simulink model "formation_with_real_uavs"  (R2022a)
settings: Solver=VariableStepAuto  StartTime=0.0  StopTime=60  RelTol=1e-3
libraries: uavutilslib x1
settings Model: Creator=klebercabral  LastModifiedBy=klebercabral
settings DebuggingCC: UnderSpecifiedDimensionMsg=warning

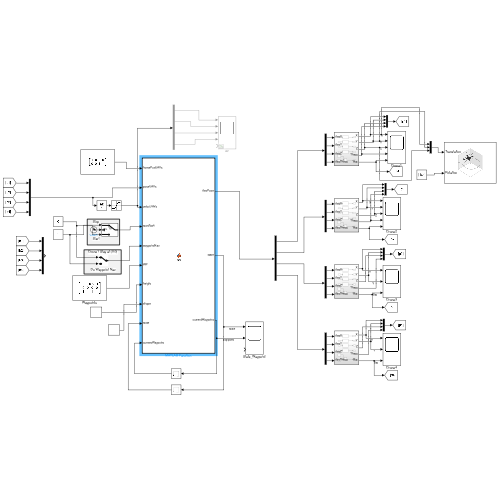
[thumbnail: Simulink's stored preview of the top-level diagram]
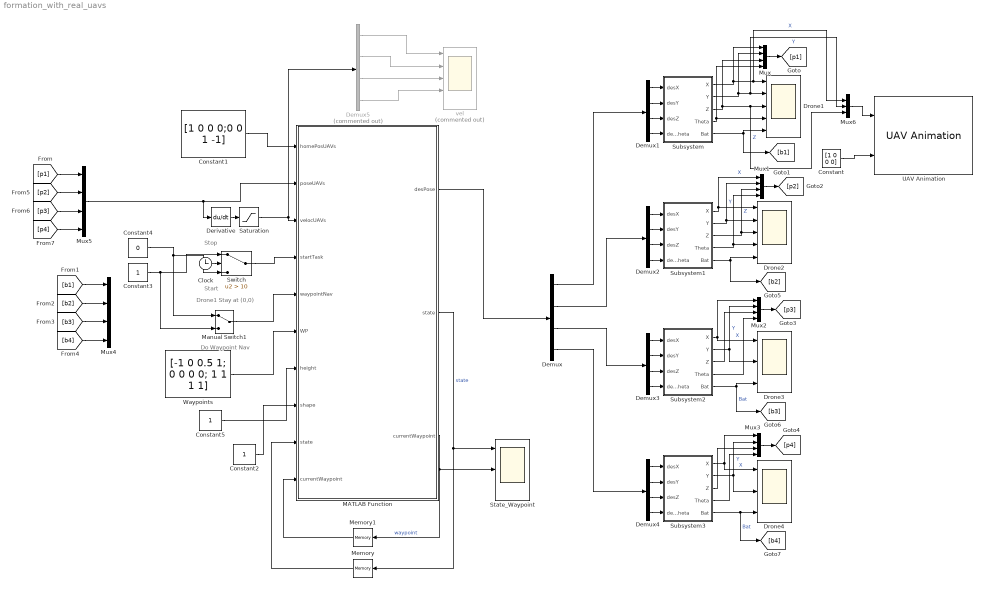
== system formation_with_real_uavs ==
  note: Stop
  note: Start
  note: Drone1 Stay at (0,0)
  note: Do Waypoint Nav
  Clock : Clock
  Constant : Constant  Value=[1 0 0 0]
  Constant1 : Constant  Value="[1 0  0  0;0  0  1 -1]"
  Constant2 : Constant
  Constant3 : Constant
  Constant4 : Constant  Value=0
  Constant5 : Constant
  Demux{,1..4} (5 alike) : Demux
  Demux5 : Demux  Commented=on
  Derivative : Derivative
  Drone1 : Scope  NumInputPorts=5
  Drone2 : Scope  NumInputPorts=5
  Drone3 : Scope  NumInputPorts=3
  Drone4 : Scope  NumInputPorts=3
  MATLAB Function : MATLAB Function  TreatAsAtomicUnit=on
  Manual Switch1 : ManualSwitch
  Memory : Memory  InitialCondition=1
  Memory1 : Memory  InitialCondition=1
  Mux{,1..5} (6 alike) : Mux
  Mux6 : Mux  Inputs=3
  Saturation : Saturate  UpperLimit=1  LowerLimit=-1
  State_Waypoint : Scope  NumInputPorts=3
  Subsystem : Subsystem
  Subsystem1 : Subsystem
  Subsystem2 : Subsystem
  Subsystem3 : Subsystem
  Switch : Switch  Criteria=u2 > Threshold  Threshold=10  SaturateOnIntegerOverflow=off  InputSameDT=off
  UAV Animation : uavutilslib/UAV Animation  UAVType=Multirotor  UAVSize=1  InertialZDirection=Up  SampleTime=-1
      settings: SourceProductBaseCode=UV
  Waypoints : Constant  Value=[-1 0 0.5 1; 0 0 0 0; 1 1 1 1]
  vel : Scope  Commented=on  NumInputPorts=5
  wires:
  Demux1/1 -> Subsystem/1(desX)
  Demux1/2 -> Subsystem/2(desY)
  Subsystem/5(Bat) -> Drone1/5, [b1]
  Subsystem1/5(Bat) -> Drone2/5, [b2]
  Subsystem2/5(Bat) -> Drone3/3, [b3]  "Bat"
  Subsystem3/5(Bat) -> [b4], Drone4/3  "Bat"
  Waypoints/1 -> MATLAB Function/6(WP)
  Mux/1 -> [p1]
  Mux1/1 -> [p2]
  Subsystem1/2(Y) -> Drone2/2, Mux1/2  "Y"
  Subsystem2/2(Y) -> Drone3/2, Mux2/2  "Y"
  Subsystem2/1(X) -> Drone3/1, Mux2/1  "X"
  Mux2/1 -> [p3]
  Mux3/1 -> [p4]
  Subsystem3/1(X) -> Drone4/1, Mux3/1  "X"
  Subsystem3/2(Y) -> Drone4/2, Mux3/2  "Y"
  [p1] -> Mux5/1
  [b1] -> Mux4/1
  [b2] -> Mux4/2
  [b4] -> Mux4/4
  [b3] -> Mux4/3
  [p2] -> Mux5/2
  [p3] -> Mux5/3
  [p4] -> Mux5/4
  Mux5/1 -> Derivative/1, MATLAB Function/2(poseUAVs)
  MATLAB Function/1(desPose) -> Demux/1
  Demux/1 -> Demux1/1
  Constant1/1 -> MATLAB Function/1(homePosUAVs)
  MATLAB Function/2(state) -> State_Waypoint/1, Memory/1  "state"
  Memory/1 -> MATLAB Function/9("state ")
  MATLAB Function/3(currentWaypoint) -> State_Waypoint/2, Memory1/1  "waypoint"
  Demux1/3 -> Subsystem/3(desZ)
  Demux1/4 -> Subsystem/4(desTheta)
  Subsystem/3(Z) -> Mux/3, Mux6/3, Drone1/3  "Z"
  Demux2/1 -> Subsystem1/1(desX)
  Demux2/2 -> Subsystem1/2(desY)
  Demux2/3 -> Subsystem1/3(desZ)
  Demux2/4 -> Subsystem1/4(desTheta)
  Demux3/1 -> Subsystem2/1(desX)
  Demux3/2 -> Subsystem2/2(desY)
  Demux3/3 -> Subsystem2/3(desZ)
  Demux3/4 -> Subsystem2/4(desTheta)
  Demux4/1 -> Subsystem3/1(desX)
  Demux4/2 -> Subsystem3/2(desY)
  Demux4/3 -> Subsystem3/3(desZ)
  Demux4/4 -> Subsystem3/4(desTheta)
  Demux/4 -> Demux4/1
  Demux/3 -> Demux3/1
  Demux/2 -> Demux2/1
  Subsystem1/3(Z) -> Drone2/3, Mux1/3  "Z"
  Subsystem2/3(Z) -> Mux2/3
  Subsystem3/3(Z) -> Mux3/3
  Subsystem/4(Theta) -> Drone1/4, Mux/4
  Subsystem1/4(Theta) -> Drone2/4, Mux1/4
  Subsystem2/4(Theta) -> Mux2/4
  Subsystem3/4(Theta) -> Mux3/4
  Subsystem/2(Y) -> Mux6/2, Drone1/2, Mux/2  "Y"
  Memory1/1 -> MATLAB Function/10("currentWaypoint ")
  Constant2/1 -> MATLAB Function/8(shape)
  Subsystem/1(X) -> Mux6/1, Drone1/1, Mux/1  "X"
  Subsystem1/1(X) -> Mux1/1, Drone2/1  "X"
  Constant/1 -> UAV Animation/2
  Mux6/1 -> UAV Animation/1
  Derivative/1 -> Saturation/1
  Saturation/1 -> MATLAB Function/3(velocUAVs), Demux5/1
  Demux5/3 -> vel/3
  Demux5/2 -> vel/2
  Demux5/4 -> vel/4
  Demux5/1 -> vel/1
  Manual Switch1/1 -> MATLAB Function/5(waypointNav)
  Switch/1 -> MATLAB Function/4(startTask)
  Constant4/1 -> Switch/3, Manual Switch1/1
  Constant3/1 -> Switch/1, Manual Switch1/2
  Constant5/1 -> MATLAB Function/7(height)
  Clock/1 -> Switch/2

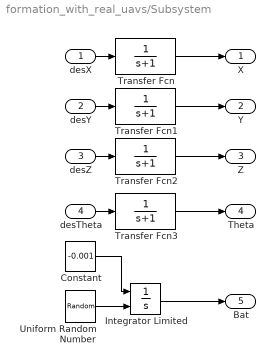
== system formation_with_real_uavs/Subsystem ==
  desX : Inport
  desY : Inport  Port=2
  desZ : Inport  Port=3
  desTheta : Inport  Port=4
  Constant : Constant  Value=-0.001
  Integrator Limited : Integrator  InitialConditionSource=external  InitialCondition=1  LimitOutput=on  UpperSaturationLimit=1  LowerSaturationLimit=0
  Transfer Fcn{,1..3} (4 alike) : TransferFcn  Denominator=[1 1]
  Uniform Random Number : UniformRandomNumber  Minimum=0.5  SampleTime=1
  X : Outport
  Y : Outport  Port=2
  Z : Outport  Port=3
  Theta : Outport  Port=4
  Bat : Outport  Port=5
  wires:
  desX/1 -> Transfer Fcn/1
  Constant/1 -> Integrator Limited/1
  Uniform Random Number/1 -> Integrator Limited/2
  Transfer Fcn/1 -> X/1
  desY/1 -> Transfer Fcn1/1
  Integrator Limited/1 -> Bat/1
  Transfer Fcn1/1 -> Y/1
  Transfer Fcn2/1 -> Z/1
  desZ/1 -> Transfer Fcn2/1
  desTheta/1 -> Transfer Fcn3/1
  Transfer Fcn3/1 -> Theta/1

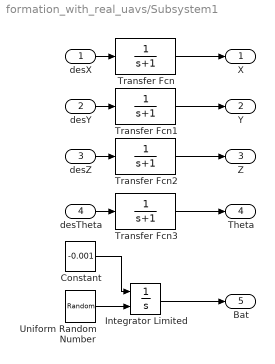
== system formation_with_real_uavs/Subsystem1 ==
  desX : Inport
  desY : Inport  Port=2
  desZ : Inport  Port=3
  desTheta : Inport  Port=4
  Constant : Constant  Value=-0.001
  Integrator Limited : Integrator  InitialConditionSource=external  InitialCondition=1  LimitOutput=on  UpperSaturationLimit=1  LowerSaturationLimit=0
  Transfer Fcn{,1..3} (4 alike) : TransferFcn  Denominator=[1 1]
  Uniform Random Number : UniformRandomNumber  Minimum=0.5  SampleTime=1
  X : Outport
  Y : Outport  Port=2
  Z : Outport  Port=3
  Theta : Outport  Port=4
  Bat : Outport  Port=5
  wires:
  Transfer Fcn3/1 -> Theta/1
  desTheta/1 -> Transfer Fcn3/1
  desZ/1 -> Transfer Fcn2/1
  Transfer Fcn2/1 -> Z/1
  Transfer Fcn1/1 -> Y/1
  Integrator Limited/1 -> Bat/1
  desY/1 -> Transfer Fcn1/1
  Transfer Fcn/1 -> X/1
  Uniform Random Number/1 -> Integrator Limited/2
  Constant/1 -> Integrator Limited/1
  desX/1 -> Transfer Fcn/1

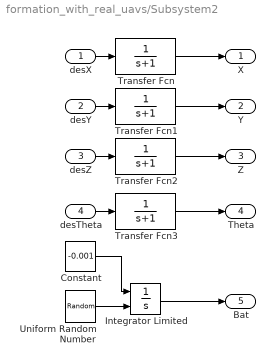
== system formation_with_real_uavs/Subsystem2 ==
  desX : Inport
  desY : Inport  Port=2
  desZ : Inport  Port=3
  desTheta : Inport  Port=4
  Constant : Constant  Value=-0.001
  Integrator Limited : Integrator  InitialConditionSource=external  InitialCondition=1  LimitOutput=on  UpperSaturationLimit=1  LowerSaturationLimit=0
  Transfer Fcn{,1..3} (4 alike) : TransferFcn  Denominator=[1 1]
  Uniform Random Number : UniformRandomNumber  Minimum=0.5  SampleTime=1
  X : Outport
  Y : Outport  Port=2
  Z : Outport  Port=3
  Theta : Outport  Port=4
  Bat : Outport  Port=5
  wires:
  desX/1 -> Transfer Fcn/1
  Constant/1 -> Integrator Limited/1
  Uniform Random Number/1 -> Integrator Limited/2
  Transfer Fcn/1 -> X/1
  desY/1 -> Transfer Fcn1/1
  Integrator Limited/1 -> Bat/1
  Transfer Fcn1/1 -> Y/1
  Transfer Fcn2/1 -> Z/1
  desZ/1 -> Transfer Fcn2/1
  desTheta/1 -> Transfer Fcn3/1
  Transfer Fcn3/1 -> Theta/1

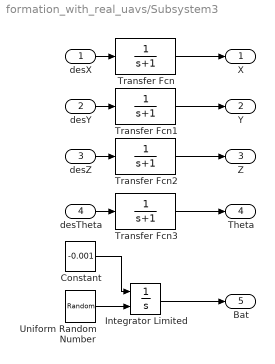
== system formation_with_real_uavs/Subsystem3 ==
  desX : Inport
  desY : Inport  Port=2
  desZ : Inport  Port=3
  desTheta : Inport  Port=4
  Constant : Constant  Value=-0.001
  Integrator Limited : Integrator  InitialConditionSource=external  InitialCondition=1  LimitOutput=on  UpperSaturationLimit=1  LowerSaturationLimit=0
  Transfer Fcn{,1..3} (4 alike) : TransferFcn  Denominator=[1 1]
  Uniform Random Number : UniformRandomNumber  Minimum=0.5  SampleTime=1
  X : Outport
  Y : Outport  Port=2
  Z : Outport  Port=3
  Theta : Outport  Port=4
  Bat : Outport  Port=5
  wires:
  Transfer Fcn3/1 -> Theta/1
  desTheta/1 -> Transfer Fcn3/1
  desZ/1 -> Transfer Fcn2/1
  Transfer Fcn2/1 -> Z/1
  Transfer Fcn1/1 -> Y/1
  Integrator Limited/1 -> Bat/1
  desY/1 -> Transfer Fcn1/1
  Transfer Fcn/1 -> X/1
  Uniform Random Number/1 -> Integrator Limited/2
  Constant/1 -> Integrator Limited/1
  desX/1 -> Transfer Fcn/1

== matlab function formation_with_real_uavs/MATLAB Function ==
  data: homePosUAVs input; poseUAVs input; velocUAVs input; startTask input; waypointNav input; WP input; height input; desPose output; shape input size=1; state output; currentWaypoint output; state input; currentWaypoint input
function [desPose, state, currentWaypoint] = fcn(...
    homePosUAVs, poseUAVs, velocUAVs,...
    startTask, waypointNav, WP, height, ...
    shape, state, currentWaypoint)

shape=max(min(shape,4), 1);
Shape = [0  1  0  0;0  0  1 -1;0  0  0  0];

switch shape
    case 1
        Shape = [
                0  1  0  0;
                0  0  1 -1;
                1  1  1  1];
    case 2
        Shape = [
                0  1  1  1;
                0  0  1 -1;
                1  1  1  1];
    case 3
        Shape = [
                0  1  0  0;
                0  0  1 -1;
                1  1  1  1];
    case 4
        Shape = [
                -1  0  0  0;
                 0  0  1 -1;
                 1  1  1  1];
end


%STATE CONDITIONS
IDLE = 1;
EXECTASK = 2;

posUAVs=reshape(poseUAVs, [], 4);
posUAVs(4,:)=[];

velUAVs=reshape(velocUAVs, [], 4);
velUAVs(4,:)=[];

desPos = [homePosUAVs;ones(1,size(homePosUAVs,2))];

epslon = 0.5;
int_range_r = 0.9;
sigma_int_range = sigma_norm(int_range_r);

kp=0.5;
N=4;
n=3;
dt=0.5;
x=posUAVs;
A=zeros(N,N);       % Ajacency Matrix
A(1,2)=1; A(1,3)=1; A(1,4)=1; 
          A(2,3)=0; A(2,4)=0; 
                    A(3,4)=0; 
A=A+A';    

switch state
    case IDLE
        %Able to run a task if one exists
        currentWaypoint=1;
        if startTask > 0 % a new task has arrived 
            state=EXECTASK;
        end


    case EXECTASK
        for i=1:N
            posi = x(1:n,i);
            posi_s = Shape(1:n,i);

            u_form = posi*0;
            u_ca = posi*0;
            u_pinning = posi*0;
            u=posi*0;

            for j=1:N
                posj = x(1:n,j);
                posj_s = Shape(1:n,j);

                if i~=j && A(i,j)~=0
                    u_form = u_form + kp*(posi - posj - posi_s + posj_s);%+ kv*(veli-velj);
                end
            end

            for j=1:N
                posj = x(1:n,j);
                diff = posj-posi;
                if i~=j && norm(diff)<int_range_r
                    %trying to avoid colisions
                    sigma_diff = sigma_norm(diff);
                    sigma_d = sigma_norm(0.9);
                    phi_alpha = rho_h(sigma_diff/sigma_int_range)*sigma_1(sigma_diff-sigma_d);
                    nij= diff/sqrt(1+epslon*norm(diff,2)^2);
                    rotNij = [sqrt(2)/2,sqrt(2)/2,0;-sqrt(2)/2,sqrt(2)/2,0;0,0,1]*nij;
                    u_ca = u_ca + 50*phi_alpha*rotNij;%nij;
                    %u_ca = u_ca + 50*phi_alpha*nij;
                    u_ca(3)=0;
                    if norm(diff)<0.8 %&& i==1
                       [th1,r1]=cart2pol(-u_form(1),-u_form(2)) ;
                       [th2,r2]=cart2pol(u_ca(1),u_ca(2));
    
                       disp([i j norm(diff) rad2deg(th1) r1 rad2deg(th2) r2])
                    end
                end
            end


%             % -------- Obstacle avoidance -------- 
%             %considering the obstacle as another agent
%             for j=1:N
%                 print=0;
% 
%                 R_k=0.6; % Radius of the 'obstacle', circle around the drone that cannot be transpassed 
%                 posj = x(1:n,j);
%                 posi(3)=1;
%                 posj(3)=1;
%                 veli=velUAVs(1:n,i);
%                 veli(3)=0;
% 
%                 d_ij = posi - posj;
%                 n_d_ij= norm(d_ij);
% 
%                 sigma_d_obs = sigma_norm(0.1); %distance from 'obstacle' surface
%                 int_range_r_obs=0.9;
%                 sigma_int_range_obs = sigma_norm(int_range_r_obs);
%                 
%                 %To run simulation faster,
%                 %avoid the calculations if the target is out of range
%                 if n_d_ij<int_range_r_obs && i~=j && n_d_ij>0.5
%                     if n_d_ij <= 1.1*R_k 
%                         u_form=u_form*0; %clear the formation control and leave just the collision avoidance
%                         print=1;
%                     end
%                     %disp([i,j,norm(diff_ij), int_range_r_obs, int_range_r_obs+0.6])
%                    
%                     mu = R_k/n_d_ij;      % obtain the vector from agent to object
%                     a_k = (d_ij)/n_d_ij;
%                     P=eye(n) - a_k * (a_k');
%                     pos_beta=mu*posi+(1-mu)*posj;         %position of beta agent (%olfati-saber modeling)
%                     vel_beta=mu*P*veli;                         %velocity of beta agent (%olfati-saber modeling)
%     
%                     diff=pos_beta-posi;
%                     sigma_diff = sigma_norm(diff);
%                     phi_beta = rho_h(sigma_diff/sigma_int_range_obs)*(sigma_1(sigma_diff-sigma_d_obs)-1);
%                     nij = diff/sqrt(1+epslon*norm(diff,2)^2);
%                     b_ik = rho_h(sigma_diff/sigma_int_range_obs);
%                     
% 
%                     col_avoid = 2.5*(phi_beta*nij + 2*b_ik*(vel_beta-veli));
%                     col_avoid(3)=0;
% 
%                     u_ca = u_ca + col_avoid;
%                 %end
% 
%                 %if print==1
%                    
%                    [th1,r1]=cart2pol(u_form(1),u_form(2)) ;
%                    [th2,r2]=cart2pol(u_ca(1),u_ca(2));
% 
%                    disp([i j n_d_ij norm(u_form) norm(u_ca) rad2deg(th1) r1 rad2deg(th2) r2])
%                    %disp([posi posj pos_beta u phi_beta*nij b_ik*(vel_beta-veli)])
%                 end
            
            %Pinning controller
            if i==1
                u_pinning = 1e0*(waypointNav*WP(1:n,currentWaypoint)-posi);% + 1e1*(WP(n+1:n+n,nextwp)-x(n+1:n+n,i));
            end
            u=-1*u_form + u_ca + u_pinning;

            desPos(1:n,i)  = x(1:n,i) + dt*u;
        end
        %desPos=x(1:n,:,2);

        %disp(norm(WP(1:n,currentWaypoint)-x(1:n,1),2))
        if norm(WP(1:n,currentWaypoint)-x(1:n,1),2)  < 0.05 
            currentWaypoint=currentWaypoint+1*waypointNav;  %if waypointNav is 0 than this variable does not change
            if currentWaypoint>size(WP,2)
                state=IDLE;
            end
        end

end
state=state(1);
desPose = reshape_pose_output(desPos(1,:),desPos(2,:),height*ones(1,4),[0 0 0 0]);
% 
% if PLOTGRAPH 
%     hold on
%     grid on 
%     plot(posUAVs(1,pin),posUAVs(2,pin),'ko','MarkerSize',25,'Linewidth',1.5); %auctioneer
%     %Plotting structures
%     for j=1:length(posTasks)
% %         plot(posTasks(1,j),posTasks(2,j), 'rx', 'MarkerSize',10)
%     end
%     valid_bids=[];
%     axis equal
% end
% 
% if PLOTGRAPH
%     h=plot(G,'XData',x(1,:),'YData',x(2,:));
%     highlight(h,T.tree);
%     drawnow
%     pause(0.1);
% end

end


function pose_output = reshape_pose_output(X_all, Y_all, Z_all, Theta_all)
pose_output=reshape([X_all; Y_all; Z_all; Theta_all],16,1);

end


function [ output ] = sigma_norm( input )
   epslon=0.5;
   output=(1/epslon)*(sqrt(1+epslon*(norm(input,2)^2))-1);
end

function [rho] = rho_h (z)
    if z >= 0 && z < 0.5
        rho=1;
    elseif z >= 0.5 && z<1
        rho= 0.5 * (1 + cos( pi * ((z-0.5)/(1-0.5))));
    else 
        rho=0;
    end
end

function [sigma1] = sigma_1(z)
    sigma1=z/(sqrt(1+norm(z)^2));
end
